simulink model "Rw02_Simulink1"  (R2015b)
settings: Solver=VariableStepAuto  StartTime=0.0  StopTime=400  RelTol=1e-3
libraries: simulink x1
settings Model: Creator=dell  LastModifiedBy=dell

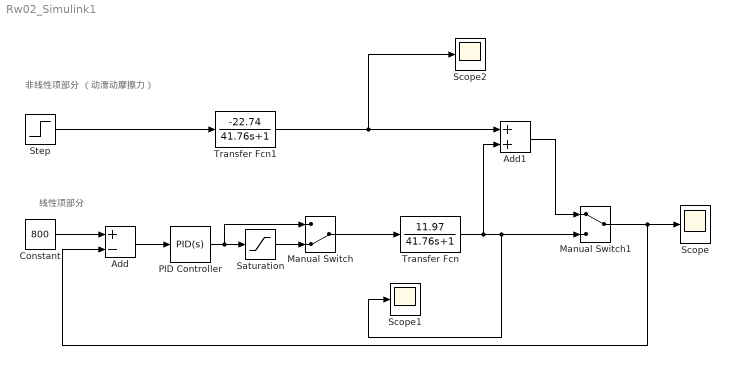
== system Rw02_Simulink1 ==
  note: 线性项部分
  note: 非线性项部分
      | （动滑动摩擦力）
  Add : Sum  Inputs=+-
  Add1 : Sum
  Constant : Constant  Value=800
  Manual Switch : ManualSwitch  CurrentSetting=0
  Manual Switch1 : ManualSwitch
  PID Controller : simulink/Continuous/PID Controller  Controller=PID  TimeDomain=Continuous-time  SampleTime=-1  IntegratorMethod=Forward Euler  FilterMethod=Forward Euler  Form=Parallel  UseFilter=on  ControllerParametersSource=internal  P=8  I=0.08  D=0  N=40  InitialConditionSource=internal  InitialConditionForIntegrator=0  InitialConditionForFilter=0  ExternalReset=none  LimitOutput=off  UpperSaturationLimit=inf  LowerSaturationLimit=-inf  LinearizeAsGain=on  AntiWindupMode=none  Kb=1  TrackingMode=off  Kt=1  PParamMin=[]  PParamMax=[]  IParamMin=[]  IParamMax=[]  DParamMin=[]  DParamMax=[]  NParamMin=[]  NParamMax=[]  KbParamMin=[]  KbParamMax=[]  KtParamMin=[]  KtParamMax=[]  POutMin=[]  POutMax=[]  IOutMin=[]  IOutMax=[]  DOutMin=[]  DOutMax=[]  NOutMin=[]  NOutMax=[]  KbOutMin=[]  KbOutMax=[]  KtOutMin=[]  KtOutMax=[]  IntegratorOutMin=[]  IntegratorOutMax=[]  FilterOutMin=[]  FilterOutMax=[]  SumOutMin=[]  SumOutMax=[]  SumI1OutMin=[]  SumI1OutMax=[]  SumI2OutMin=[]  SumI2OutMax=[]  SumI3OutMin=[]  SumI3OutMax=[]  SumDOutMin=[]  SumDOutMax=[]  SaturationOutMin=[]  SaturationOutMax=[]  IntegratorContinuousStateAttributes=''  IntegratorStateMustResolveToSignalObject=off  IntegratorRTWStateStorageClass=Auto  FilterContinuousStateAttributes=''  FilterStateMustResolveToSignalObject=off  FilterRTWStateStorageClass=Auto  DifferentiatorICPrevScaledInput=0  DifferentiatorOutMin=[]  DifferentiatorOutMax=[]
  Saturation : Saturate  UpperLimit=127  LowerLimit=-127
  Scope : Scope
  Scope1 : Scope
  Scope2 : Scope
  Step : Step  Time=0  SampleTime=0
  Transfer Fcn : TransferFcn  Numerator=[11.97]  Denominator=[41.76 1]
  Transfer Fcn1 : TransferFcn  Numerator=[-22.74]  Denominator=[41.76 1]
  wires:
  Saturation/1 -> Manual Switch/2
  Constant/1 -> Add/1
  Add/1 -> PID Controller/1
  PID Controller/1 -> Manual Switch/1, Saturation/1
  Manual Switch/1 -> Transfer Fcn/1
  Step/1 -> Transfer Fcn1/1
  Transfer Fcn1/1 -> Scope2/1, Add1/1
  Transfer Fcn/1 -> Add1/2, Scope1/1, Manual Switch1/2
  Add1/1 -> Manual Switch1/1
  Manual Switch1/1 -> Add/2, Scope/1
